simulink subsystem "Day3_Scenario_2"  (R2024a)
settings: Solver=VariableStepAuto  StartTime=0.0  StopTime=10.0  RelTol=1e-3
libraries: CarMaker4SL x8, slpidlib x1
settings Model: Creator=junhyung.cha  LastModifiedBy=User

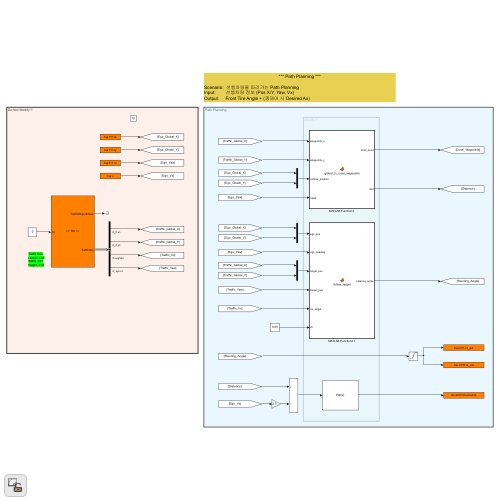
[thumbnail: Simulink's stored preview of the top-level diagram]
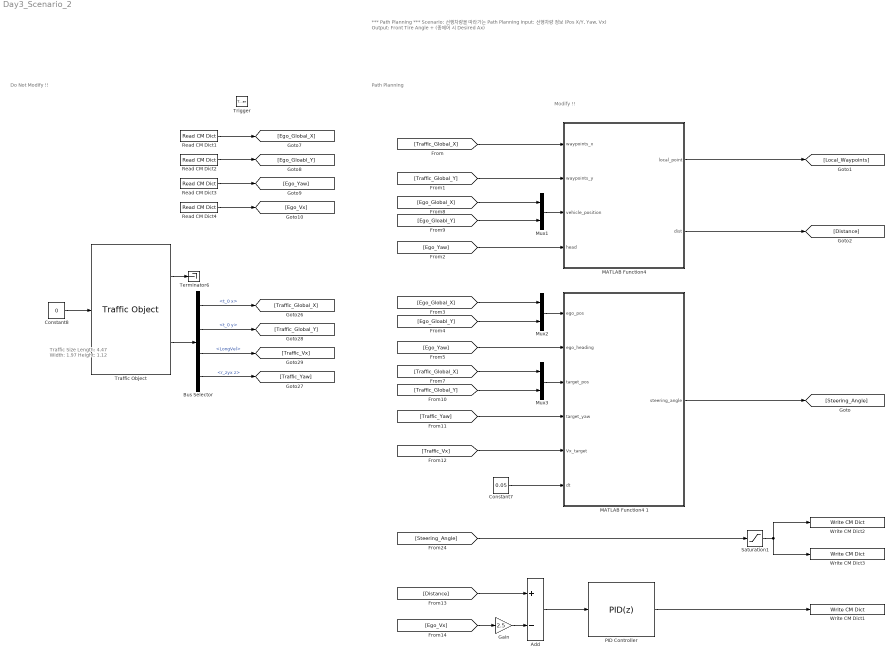
== system Day3_Scenario_2 ==
  note: Path Planning
  note: Do Not Modify !!
  note: Modify !!
  note: *** Path Planning ***
      |
      | Scenario: 선행차량을 따라가는 Path Planning
      | Input: 선행차량 정보 (Pos X/Y, Yaw, Vx)
      | Output: Front Tire Angle + (종제어 시 Desired Ax)
  note: Traffic Size
      | Length: 4.47
      | Width: 1.97
      | Height: 1.12
  Trigger : TriggerPort  TriggerType=function-call  VariantControl=(inherit)
  Add : Sum  Inputs=+-
  Bus Selector : BusSelector  OutputSignals=t_0 x,t_0 y,LongVel,r_zyx z
  Constant7 : Constant  Value=0.05
  Constant8 : Constant  Value=0
  Gain : Gain  Gain=2.5
  "MATLAB Function4 " : MATLAB Function  TreatAsAtomicUnit=on
  MATLAB Function4 1 : MATLAB Function  TreatAsAtomicUnit=on
  Mux1 : Mux  Inputs=2
  Mux2 : Mux  Inputs=2
  Mux3 : Mux  Inputs=2
  PID Controller : slpidlib/PID Controller  Controller=PID  Form=Parallel  TimeDomain=Discrete-time  UseExternalTs=off  SampleTime=-1  IntegratorMethod=Forward Euler  FilterMethod=Forward Euler  ControllerParametersSource=internal  P=3  I=0.01  UseKiTs=off  D=0  UseExternalDerivativeSource=off  N=100  UseFilter=on  TunerSelectOption=Transfer Function Based (PID Tuner App)  InitialConditionSource=internal  InitialConditionForIntegrator=0  InitialConditionForFilter=0  DifferentiatorICPrevScaledInput=0  ExternalReset=none  TrackingMode=off  Kt=1  LimitOutput=off  SatLimitsSource=internal  UpperSaturationLimit=inf  LowerSaturationLimit=-inf  LinearizeAsGain=on  AntiWindupMode=none  Kb=1  LimitIntegrator=off  UpperIntegratorSaturationLimit=inf  LowerIntegratorSaturationLimit=-inf  POutMin=[]  POutMax=[]  IOutMin=[]  IOutMax=[]  DOutMin=[]  DOutMax=[]  NOutMin=[]  NOutMax=[]  SumOutMin=[]  SumOutMax=[]  SaturationOutMin=[]  SaturationOutMax=[]  PParamMin=[]  PParamMax=[]  IParamMin=[]  IParamMax=[]  DParamMin=[]  DParamMax=[]  NParamMin=[]  NParamMax=[]  KbParamMin=[]  KbParamMax=[]  KtParamMin=[]  KtParamMax=[]  KbOutMin=[]  KbOutMax=[]  KtOutMin=[]  KtOutMax=[]  IntegratorOutMin=[]  IntegratorOutMax=[]  FilterOutMin=[]  FilterOutMax=[]  SumI1OutMin=[]  SumI1OutMax=[]  SumI2OutMin=[]  SumI2OutMax=[]  SumI3OutMin=[]  SumI3OutMax=[]  SumI4OutMin=[]  SumI4OutMax=[]  SumDOutMin=[]  SumDOutMax=[]  DifferentiatorOutMin=[]  DifferentiatorOutMax=[]  FilterDiffOutCoefMin=[]  FilterDiffOutCoefMax=[]  ReciprocalOutMin=[]  ReciprocalOutMax=[]  SumDenOutMin=[]  SumDenOutMax=[]  SumNumOutMin=[]  SumNumOutMax=[]  DivideOutMin=[]  DivideOutMax=[]  UdiffTsProdOutMin=[]  UdiffTsProdOutMax=[]  NTsProdOutMin=[]  NTsProdOutMax=[]  UintegralTsProdOutMin=[]  UintegralTsProdOutMax=[]  UngainTsProdOutMin=[]  UngainTsProdOutMax=[]  ClampingZeroOutDataTypeStr=Inherit: Inherit via back propagation  ClampingZeroOutMin=[]  ClampingZeroOutMax=[]  FilterDenConstantOutDataTypeStr=Inherit: Inherit via back propagation  FilterDenConstantOutMin=[]  FilterDenConstantOutMax=[]  PCopyOutDataTypeStr=Inherit: Inherit via back propagation  PCopyOutMin=[]  PCopyOutMax=[]  NCopyOutDataTypeStr=Inherit: Inherit via back propagation  NCopyOutMin=[]  NCopyOutMax=[]  IntegratorContinuousStateAttributes=''  IntegratorStateMustResolveToSignalObject=off  IntegratorRTWStateStorageClass=Auto  FilterContinuousStateAttributes=''  FilterStateMustResolveToSignalObject=off  FilterRTWStateStorageClass=Auto  ParallelPVariant=InternalParameters  IdealPVariant=Disabled  IVariant=InternalParameters  DVariant=InternalParameters  IntegratorVariant=Discrete  SatVariant=Disabled  AWVariant=Passthrough  PCopyVariant=Disabled  TRVariant=Disabled  FdbkBlocksVariant=Forward  IdealPFdbkVariant=Disabled  SatFdbkVariant=Disabled  DerivativeFilterVariant=ForwardEulerFilter  NVariant=InternalParameters  NCopyVariant=Disabled  FilterICVariant=InternalICsFilter  IntegratorICVariant=InternalICs  ExternalResetVariant=Disabled  TRSumVariant=Passthrough  SumFdbkVariant=Disabled  SumVariant=Sum_PID  TsampFilterVariant=InternalTs  TsampNgainVariant=Passthrough  TsampIntegralVariant=Disabled_SignalSpec  ExternalSaturationOutDataTypeStr=Inherit: Same as second input  DerivativeSourceVariant=ErrorSignal
  Read CM Dict1 : CarMaker4SL/Read CM Dict  xname=Car.Fr1.tx  xsync=off  xstime=Inherited
  Read CM Dict2 : CarMaker4SL/Read CM Dict  xname=Car.Fr1.ty  xsync=off  xstime=Inherited
  Read CM Dict3 : CarMaker4SL/Read CM Dict  xname=Car.Fr1.rz  xsync=off  xstime=Inherited
  Read CM Dict4 : CarMaker4SL/Read CM Dict  xname=Car.v  xsync=off  xstime=Inherited
  Saturation1 : Saturate  UpperLimit=pi/6  LowerLimit=-pi/6
  Terminator6 : Terminator
  Traffic Object : CarMaker4SL/Traffic Object  xname=T00  ximode=Traffic Id  xstime=Inherited
      settings: SourceProductName=CarMaker4SL
  Write CM Dict1 : CarMaker4SL/Write CM Dict  xname=AccelCtrl.DesiredAx  xsync=off
  Write CM Dict2 : CarMaker4SL/Write CM Dict  xname=Car.CFL.rz_ext  xsync=off
  Write CM Dict3 : CarMaker4SL/Write CM Dict  xname=Car.CFR.rz_ext  xsync=off
  wires:
  Read CM Dict4/1 -> [Ego_Vx]
  Saturation1/1 -> Write CM Dict3/1, Write CM Dict2/1
  Read CM Dict3/1 -> [Ego_Yaw]
  Read CM Dict1/1 -> [Ego_Global_X]
  Read CM Dict2/1 -> [Ego_Gloabl_Y]
  [Steering_Angle] -> Saturation1/1
  Traffic Object/2 -> Bus Selector/1
  Constant8/1 -> Traffic Object/1
  Bus Selector/4 -> [Traffic_Yaw]  "<r_zyx z>"
  Bus Selector/3 -> [Traffic_Vx]  "<LongVel>"
  Traffic Object/1 -> Terminator6/1
  Bus Selector/2 -> [Traffic_Global_Y]  "<t_0 y>"
  Bus Selector/1 -> [Traffic_Global_X]  "<t_0 x>"
  [Traffic_Global_X] -> "MATLAB Function4 "/1(waypoints_x)
  [Traffic_Global_Y] -> "MATLAB Function4 "/2(waypoints_y)
  [Ego_Gloabl_Y] -> Mux1/2
  Mux1/1 -> "MATLAB Function4 "/3(vehicle_position)
  [Ego_Global_X] -> Mux1/1
  [Ego_Yaw] -> "MATLAB Function4 "/4(head)
  "MATLAB Function4 "/1(local_point) -> [Local_Waypoints]
  "MATLAB Function4 "/2(dist) -> [Distance]
  [Ego_Global_X] -> Mux2/1
  [Ego_Gloabl_Y] -> Mux2/2
  Mux2/1 -> MATLAB Function4 1/1(ego_pos)
  [Ego_Yaw] -> MATLAB Function4 1/2(ego_heading)
  [Traffic_Global_X] -> Mux3/1
  [Traffic_Global_Y] -> Mux3/2
  [Traffic_Yaw] -> MATLAB Function4 1/4(target_yaw)
  Mux3/1 -> MATLAB Function4 1/3(target_pos)
  [Traffic_Vx] -> MATLAB Function4 1/5(Vx_target)
  Constant7/1 -> MATLAB Function4 1/6(dt)
  MATLAB Function4 1/1(steering_angle) -> [Steering_Angle]
  [Distance] -> Add/1
  [Ego_Vx] -> Gain/1
  Add/1 -> PID Controller/1
  PID Controller/1 -> Write CM Dict1/1
  Gain/1 -> Add/2

== matlab function Day3_Scenario_2/MATLAB Function4  ==
  settings: sampleTime=0.1
  data: waypoints_x input; waypoints_y input; local_point output; vehicle_position input; head input; dist output
function [local_point,dist]  = global_to_local_waypoints(waypoints_x,waypoints_y, vehicle_position, head)
    [local_point,dist] = deal(0);
end

== matlab function Day3_Scenario_2/MATLAB Function4 1 ==
  settings: sampleTime=0.1
  data: ego_pos input; ego_heading input; steering_angle output; target_pos input; target_yaw input; Vx_target input; dt input
function steering_angle = follow_target(ego_pos, ego_heading, target_pos, target_yaw, Vx_target, dt)
%#codegen
persistent stopped

% 초기화
if isempty(stopped)
    stopped = false;
end

L = 4.0;
epsilon = 1e-3;
lookahead_time = 3.0;

% Ego 및 Target
x_ego = ego_pos(1);
y_ego = ego_pos(2);
x_t = target_pos(1);
y_t = target_pos(2);

% Local 변환
dx = x_t - x_ego;
dy = y_t - y_ego;

cos_yaw = cos(-ego_heading);
sin_yaw = sin(-ego_heading);
R = [cos_yaw, -sin_yaw;
     sin_yaw,  cos_yaw];

local_pos = R * [dx; dy];
x_local = local_pos(1);
y_local = local_pos(2);
dist = sqrt(x_local^2 + y_local^2);

% 도달 조건 만족 시 정지 상태 진입
if dist < 1.0
    stopped = true;
    steering_angle = 0;
    return;
end

% 정상 Pure Pursuit 제어
denominator = x_local^2 + y_local^2 + epsilon;
steering_angle = atan2(2 * L * y_local, denominator);

end
